simulink model "MVB"  (R2013b)
settings: Solver=ode45  StartTime=0.0  StopTime=2e-5  RelTol=1e-3
libraries: simulink x2
settings Model: Creator=qiji  LastModifiedBy=qiji

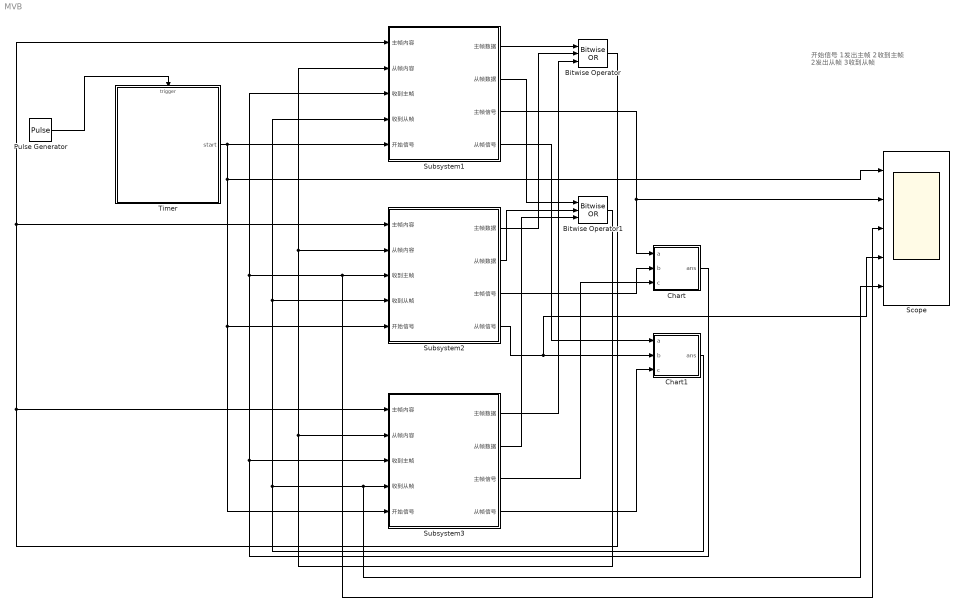
== system MVB ==
  note: 开始信号
      | 1发出主帧
      | 2收到主帧
      | 2发出从帧
      | 3收到从帧
  Bitwise Operator : simulink/Logic and Bit Operations/Bitwise Operator  logicop=OR  UseBitMask=off  NumInputPorts=3  BitMask=bin2dec('11011001')  BitMaskRealWorld=Stored Integer
  Bitwise Operator1 : simulink/Logic and Bit Operations/Bitwise Operator  logicop=OR  UseBitMask=off  NumInputPorts=3  BitMask=bin2dec('11011001')  BitMaskRealWorld=Stored Integer
  Chart : Stateflow chart  TreatAsAtomicUnit=on
  Chart1 : Stateflow chart  TreatAsAtomicUnit=on
  Pulse Generator : DiscretePulseGenerator  PulseType=Time based  Period=1e-7  PulseWidth=50
  Scope : Scope  NumInputPorts=5
      settings: YMin=-5~-5~-5~-5~-5  YMax=5~5~5~5~5
  Subsystem1 : Subsystem
  Subsystem2 : Subsystem
  Subsystem3 : Subsystem
  Timer : Stateflow chart  TreatAsAtomicUnit=on
  wires:
  Pulse Generator/1 -> Timer/Trigger
  Timer/1(start) -> Scope/1, Subsystem3/5(开始信号), Subsystem2/5(开始信号), Subsystem1/5(开始信号)
  Subsystem1/1(主帧数据) -> Bitwise Operator/1
  Subsystem2/1(主帧数据) -> Bitwise Operator/2
  Subsystem3/1(主帧数据) -> Bitwise Operator/3
  Bitwise Operator/1 -> Subsystem1/1(主帧内容), Subsystem2/1(主帧内容), Subsystem3/1(主帧内容)
  Chart/1(ans) -> Subsystem3/3(收到主帧), Subsystem1/3(收到主帧), Scope/3, Subsystem2/3(收到主帧)
  Chart1/1(ans) -> Subsystem2/4(收到从帧), Subsystem1/4(收到从帧), Scope/5, Subsystem3/4(收到从帧)
  Subsystem1/2(从帧数据) -> Bitwise Operator1/1
  Subsystem2/2(从帧数据) -> Bitwise Operator1/2
  Subsystem3/2(从帧数据) -> Bitwise Operator1/3
  Bitwise Operator1/1 -> Subsystem3/2(从帧内容), Subsystem1/2(从帧内容), Subsystem2/2(从帧内容)
  Subsystem1/3(主帧信号) -> Scope/2, Chart/1(a)
  Subsystem2/3(主帧信号) -> Chart/2(b)
  Subsystem3/3(主帧信号) -> Chart/3(c)
  Subsystem1/4(从帧信号) -> Chart1/1(a)
  Subsystem2/4(从帧信号) -> Scope/4, Chart1/2(b)
  Subsystem3/4(从帧信号) -> Chart1/3(c)

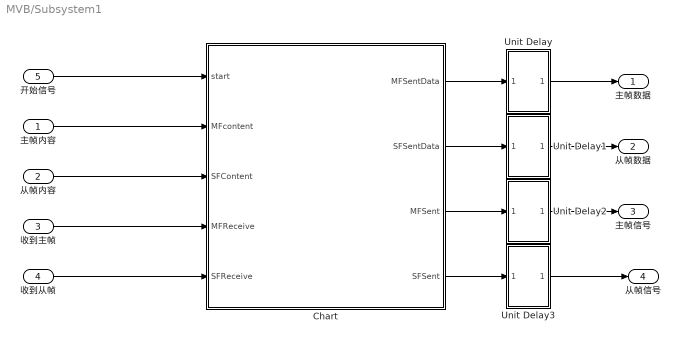
== system MVB/Subsystem1 ==
  主帧内容 : Inport
  从帧内容 : Inport  Port=2
  收到主帧 : Inport  Port=3
  收到从帧 : Inport  Port=4
  开始信号 : Inport  Port=5
  Chart : Stateflow chart  TreatAsAtomicUnit=on
  Unit Delay : Subsystem
  Unit Delay1 : Subsystem
  Unit Delay2 : Subsystem
  Unit Delay3 : Subsystem
  主帧数据 : Outport
  从帧数据 : Outport  Port=2
  主帧信号 : Outport  Port=3
  从帧信号 : Outport  Port=4
  wires:
  从帧内容/1 -> Chart/3(SFContent)
  收到主帧/1 -> Chart/4(MFReceive)
  收到从帧/1 -> Chart/5(SFReceive)
  Chart/2(SFSentData) -> Unit Delay1/1(In1)
  主帧内容/1 -> Chart/2(MFcontent)
  Chart/1(MFSentData) -> Unit Delay/1(In1)
  Chart/4(SFSent) -> Unit Delay3/1(In1)
  Chart/3(MFSent) -> Unit Delay2/1(In1)
  开始信号/1 -> Chart/1(start)
  Unit Delay/1(Out1) -> 主帧数据/1
  Unit Delay1/1(Out1) -> 从帧数据/1
  Unit Delay2/1(Out1) -> 主帧信号/1
  Unit Delay3/1(Out1) -> 从帧信号/1

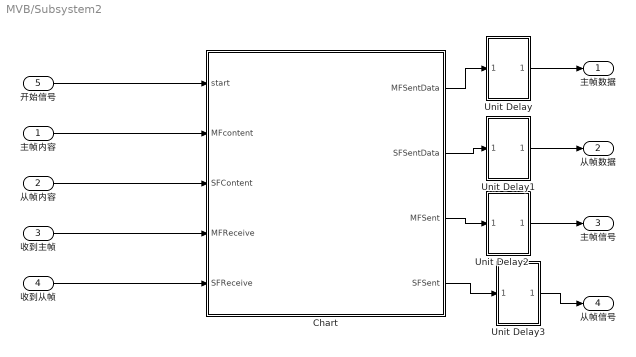
== system MVB/Subsystem2 ==
  主帧内容 : Inport
  从帧内容 : Inport  Port=2
  收到主帧 : Inport  Port=3
  收到从帧 : Inport  Port=4
  开始信号 : Inport  Port=5
  Chart : Stateflow chart  TreatAsAtomicUnit=on
  Unit Delay : Subsystem
  Unit Delay1 : Subsystem
  Unit Delay2 : Subsystem
  Unit Delay3 : Subsystem
  主帧数据 : Outport
  从帧数据 : Outport  Port=2
  主帧信号 : Outport  Port=3
  从帧信号 : Outport  Port=4
  wires:
  从帧内容/1 -> Chart/3(SFContent)
  收到主帧/1 -> Chart/4(MFReceive)
  收到从帧/1 -> Chart/5(SFReceive)
  Chart/2(SFSentData) -> Unit Delay1/1(In1)
  主帧内容/1 -> Chart/2(MFcontent)
  Chart/1(MFSentData) -> Unit Delay/1(In1)
  Chart/4(SFSent) -> Unit Delay3/1(In1)
  Chart/3(MFSent) -> Unit Delay2/1(In1)
  开始信号/1 -> Chart/1(start)
  Unit Delay/1(Out1) -> 主帧数据/1
  Unit Delay1/1(Out1) -> 从帧数据/1
  Unit Delay2/1(Out1) -> 主帧信号/1
  Unit Delay3/1(Out1) -> 从帧信号/1

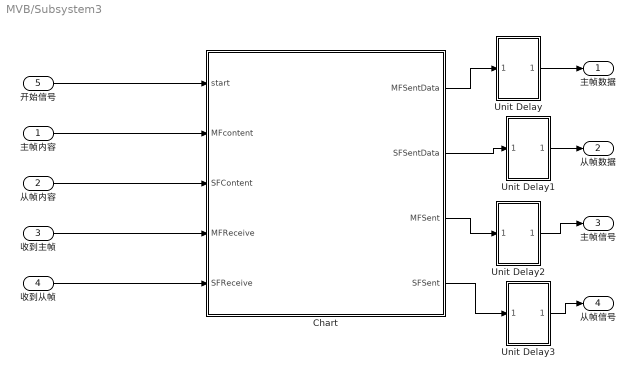
== system MVB/Subsystem3 ==
  主帧内容 : Inport
  从帧内容 : Inport  Port=2
  收到主帧 : Inport  Port=3
  收到从帧 : Inport  Port=4
  开始信号 : Inport  Port=5
  Chart : Stateflow chart  TreatAsAtomicUnit=on
  Unit Delay : Subsystem
  Unit Delay1 : Subsystem
  Unit Delay2 : Subsystem
  Unit Delay3 : Subsystem
  主帧数据 : Outport
  从帧数据 : Outport  Port=2
  主帧信号 : Outport  Port=3
  从帧信号 : Outport  Port=4
  wires:
  从帧内容/1 -> Chart/3(SFContent)
  收到主帧/1 -> Chart/4(MFReceive)
  收到从帧/1 -> Chart/5(SFReceive)
  Chart/2(SFSentData) -> Unit Delay1/1(In1)
  主帧内容/1 -> Chart/2(MFcontent)
  Chart/1(MFSentData) -> Unit Delay/1(In1)
  Chart/4(SFSent) -> Unit Delay3/1(In1)
  Chart/3(MFSent) -> Unit Delay2/1(In1)
  开始信号/1 -> Chart/1(start)
  Unit Delay/1(Out1) -> 主帧数据/1
  Unit Delay1/1(Out1) -> 从帧数据/1
  Unit Delay2/1(Out1) -> 主帧信号/1
  Unit Delay3/1(Out1) -> 从帧信号/1

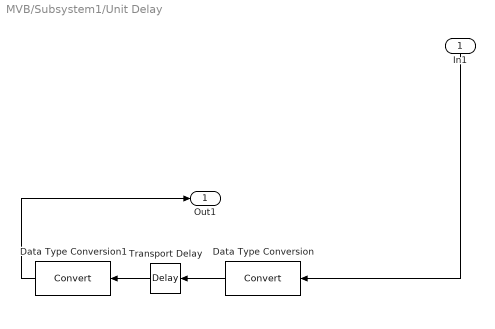
== system MVB/Subsystem1/Unit Delay ==
  In1 : Inport
  Data Type Conversion : DataTypeConversion
  Data Type Conversion1 : DataTypeConversion
  Transport Delay : TransportDelay  DelayTime=1e-7
  Out1 : Outport
  wires:
  In1/1 -> Data Type Conversion/1
  Data Type Conversion/1 -> Transport Delay/1
  Transport Delay/1 -> Data Type Conversion1/1
  Data Type Conversion1/1 -> Out1/1

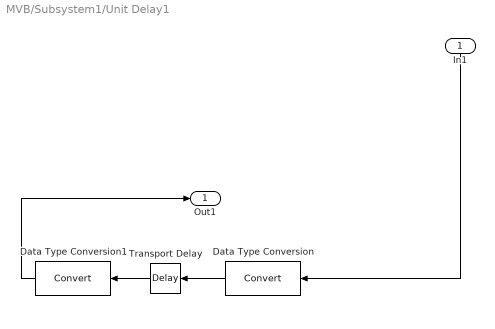
== system MVB/Subsystem1/Unit Delay1 ==
  In1 : Inport
  Data Type Conversion : DataTypeConversion
  Data Type Conversion1 : DataTypeConversion
  Transport Delay : TransportDelay  DelayTime=1e-7
  Out1 : Outport
  wires:
  In1/1 -> Data Type Conversion/1
  Data Type Conversion/1 -> Transport Delay/1
  Transport Delay/1 -> Data Type Conversion1/1
  Data Type Conversion1/1 -> Out1/1

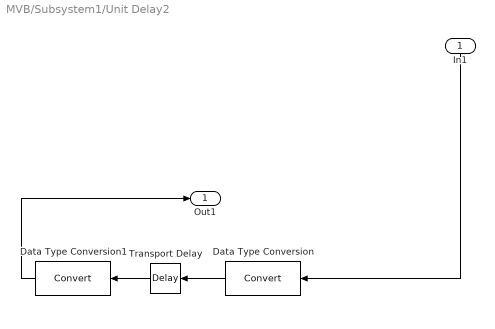
== system MVB/Subsystem1/Unit Delay2 ==
  In1 : Inport
  Data Type Conversion : DataTypeConversion
  Data Type Conversion1 : DataTypeConversion
  Transport Delay : TransportDelay  DelayTime=1e-7
  Out1 : Outport
  wires:
  In1/1 -> Data Type Conversion/1
  Data Type Conversion/1 -> Transport Delay/1
  Transport Delay/1 -> Data Type Conversion1/1
  Data Type Conversion1/1 -> Out1/1

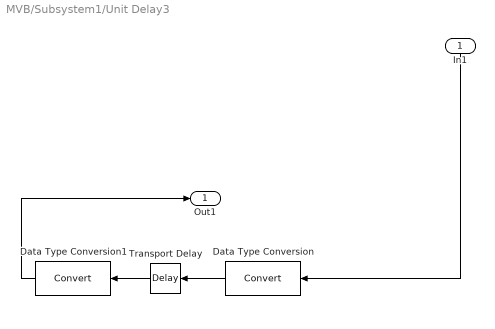
== system MVB/Subsystem1/Unit Delay3 ==
  In1 : Inport
  Data Type Conversion : DataTypeConversion
  Data Type Conversion1 : DataTypeConversion
  Transport Delay : TransportDelay  DelayTime=1e-7
  Out1 : Outport
  wires:
  In1/1 -> Data Type Conversion/1
  Data Type Conversion/1 -> Transport Delay/1
  Transport Delay/1 -> Data Type Conversion1/1
  Data Type Conversion1/1 -> Out1/1

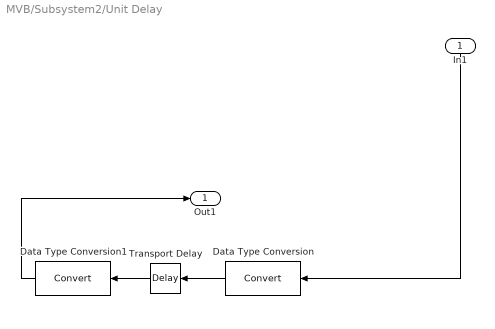
== system MVB/Subsystem2/Unit Delay ==
  In1 : Inport
  Data Type Conversion : DataTypeConversion
  Data Type Conversion1 : DataTypeConversion
  Transport Delay : TransportDelay  DelayTime=1e-7
  Out1 : Outport
  wires:
  In1/1 -> Data Type Conversion/1
  Data Type Conversion/1 -> Transport Delay/1
  Transport Delay/1 -> Data Type Conversion1/1
  Data Type Conversion1/1 -> Out1/1

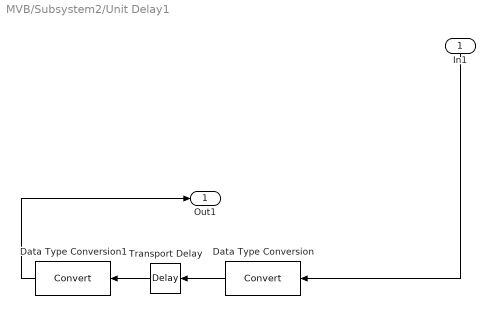
== system MVB/Subsystem2/Unit Delay1 ==
  In1 : Inport
  Data Type Conversion : DataTypeConversion
  Data Type Conversion1 : DataTypeConversion
  Transport Delay : TransportDelay  DelayTime=1e-7
  Out1 : Outport
  wires:
  In1/1 -> Data Type Conversion/1
  Data Type Conversion/1 -> Transport Delay/1
  Transport Delay/1 -> Data Type Conversion1/1
  Data Type Conversion1/1 -> Out1/1

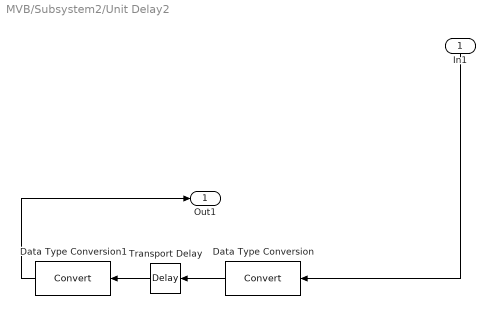
== system MVB/Subsystem2/Unit Delay2 ==
  In1 : Inport
  Data Type Conversion : DataTypeConversion
  Data Type Conversion1 : DataTypeConversion
  Transport Delay : TransportDelay  DelayTime=1e-7
  Out1 : Outport
  wires:
  In1/1 -> Data Type Conversion/1
  Data Type Conversion/1 -> Transport Delay/1
  Transport Delay/1 -> Data Type Conversion1/1
  Data Type Conversion1/1 -> Out1/1

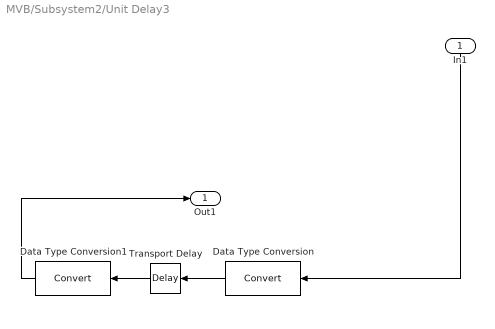
== system MVB/Subsystem2/Unit Delay3 ==
  In1 : Inport
  Data Type Conversion : DataTypeConversion
  Data Type Conversion1 : DataTypeConversion
  Transport Delay : TransportDelay  DelayTime=1e-7
  Out1 : Outport
  wires:
  In1/1 -> Data Type Conversion/1
  Data Type Conversion/1 -> Transport Delay/1
  Transport Delay/1 -> Data Type Conversion1/1
  Data Type Conversion1/1 -> Out1/1

== system MVB/Subsystem3/Unit Delay ==
  In1 : Inport
  Data Type Conversion : DataTypeConversion
  Data Type Conversion1 : DataTypeConversion
  Transport Delay : TransportDelay  DelayTime=1e-7
  Out1 : Outport
  wires:
  In1/1 -> Data Type Conversion/1
  Data Type Conversion/1 -> Transport Delay/1
  Transport Delay/1 -> Data Type Conversion1/1
  Data Type Conversion1/1 -> Out1/1

== system MVB/Subsystem3/Unit Delay1 ==
  In1 : Inport
  Data Type Conversion : DataTypeConversion
  Data Type Conversion1 : DataTypeConversion
  Transport Delay : TransportDelay  DelayTime=1e-7
  Out1 : Outport
  wires:
  In1/1 -> Data Type Conversion/1
  Data Type Conversion/1 -> Transport Delay/1
  Transport Delay/1 -> Data Type Conversion1/1
  Data Type Conversion1/1 -> Out1/1

== system MVB/Subsystem3/Unit Delay2 ==
  In1 : Inport
  Data Type Conversion : DataTypeConversion
  Data Type Conversion1 : DataTypeConversion
  Transport Delay : TransportDelay  DelayTime=1e-7
  Out1 : Outport
  wires:
  In1/1 -> Data Type Conversion/1
  Data Type Conversion/1 -> Transport Delay/1
  Transport Delay/1 -> Data Type Conversion1/1
  Data Type Conversion1/1 -> Out1/1

== system MVB/Subsystem3/Unit Delay3 ==
  In1 : Inport
  Data Type Conversion : DataTypeConversion
  Data Type Conversion1 : DataTypeConversion
  Transport Delay : TransportDelay  DelayTime=1e-7
  Out1 : Outport
  wires:
  In1/1 -> Data Type Conversion/1
  Data Type Conversion/1 -> Transport Delay/1
  Transport Delay/1 -> Data Type Conversion1/1
  Data Type Conversion1/1 -> Out1/1

== stateflow chart MVB/Timer ==
  state startTimer
  state cycle
  (default) -> startTimer
  startTimer -> cycle : {
      | cycleCount = 1000;
      | }
  (junction 5) -> cycle [order 2]
  (junction 5) -> cycle [order 1] : [cycleCount>=1000]{cycleCount=0;start = 1;}
  cycle -> (junction 5) : pulse
      | {
      | cycleCount++;
      | start = 0;
      |  }
  data: cycleCount local uint32; start output uint8
  events: pulse input RISING_EDGE_EVENT

== stateflow chart MVB/Subsystem1/Chart ==
  state startState
  state SEquipment
    state waitMF
    state judge
    state destin
    state source
    state waitSF
    state sendSF
    state checkSF
    state judgeSF
    state storeSF
    (default) -> waitMF
    waitMF -> judge : [MFReceive == 1]
        | {
        | MFaddr = MFcontent;
        | }
    judge -> destin [order 3]
    judge -> source [order 1] : [MFaddr == (logicAddr >> 12 )]
    destin -> waitSF : {
        | SFCount = 0;
        | }
    source -> sendSF : {
        | SFSent = 1;
        | SFSentData = getCongData();
        | Wait4us = 0;
        | }
    waitSF -> judgeSF [order 1] : [SFCount <= 42]
        | {
        | SFCount++;
        | }
    waitSF -> checkSF [order 2]
    judgeSF -> waitSF [order 2]
    (junction 178) -> sendSF
    sendSF -> (junction 178) [order 1] : [Wait4us <= 4]
        | {
        | Wait4us++;
        | }
    checkSF -> storeSF [order 1] : [SFReceive == 1]
        | {
        | SFCount = 0;
        | store[storeIndex] = SFContent;
        | storeIndex++;
        | }
    judgeSF -> checkSF [order 1] : [SFReceive==1]
  state MEquipment
    state waitStart
    state beforeSend
    state sendMF
    (default) -> waitStart
    waitStart -> beforeSend : [start==1]
        | {
        | MFSent = 0;
        | SFSent = 0;
        | }
    beforeSend -> MEquipment [order 2]
    beforeSend -> sendMF [order 1] : [MFNum>0]
        | {
        | MFSent = 1;
        | MFNum--;
        | MFSentData = MFT[i];
        | }
  note: 从帧和主帧已经发出，
      | 等待下一轮周期
  state r = getAddr(f_code, addr, addrReal) [function]
    (default) -> (junction 59) : {
        | r = addrReal;
        | r += (addr << 12);
        | r += (f_code << 24);
        | }
  state init [function]
    (default) -> (junction 4) : {
        | isMaster[1] = true;
        | isMaster[2] = true;
        | isMaster[3] = false;
        | isMaster[4] = false;
        | MFNum = 2;
        | i=1;
        | MFT[1] = getMF(0, 2);
        | MFT[2] = getMF(0, 3);
        | logicAddr = getAddr(0, 1, 5);
        | store[1] = 11;
        | store[2] = 22;
        | store[3] = 33;
        | store[4] = 44;
        | store[5] = 55;
        | store[6] = 66;
        | storeIndex = 7;
        | MFSent = 0;
        | SFSent = 0;
        | }
  state r = getMF(f_code, addr) [function]
    (default) -> (junction 18) : {
        | r = f_code<<12;
        | r += addr;
        | }
  state r = getCongData [function]
    (default) -> (junction 80) : {
        | r = store[logicAddr & 4095]
        | }
  (default) -> startState : {init();}
  startState -> SEquipment [order 2] : {
      | MFSent = 0;
      | SFSent = 0;
      | }
  startState -> MEquipment [order 1] : [isMaster[i]==true]
  (junction 139) -> startState : {
      | i++;
      | }
  sendMF -> (junction 139) : {
      | MFSent = 0;
      | MFSentData = 0;
      | }
  storeSF -> (junction 139)
  sendSF -> (junction 139) [order 2] : {
      | SFSent = 0;
      | }
  checkSF -> (junction 139) [order 2]
  judge -> MEquipment [order 2] : [isMaster[i]==true]
  data: r function_output double; f_code function_input double; addr function_input double; addrReal function_input double; f_code function_input double; addr function_input double; r function_output double; r function_output double; isMaster local boolean size=100; start input uint8; MFT local uint32 size=10; MFNum local uint8; i local uint8; MFSentData output uint32; MFcontent input uint32; logicAddr local uint32; store local uint32 size=100; SFSentData output uint32; storeIndex local uint32; SFContent input uint32; MFaddr local uint32; MFSent output uint8; SFSent output uint8; MFReceive input uint8; SFReceive input uint8; Wait4us local uint32; SFCount local uint32

== stateflow chart MVB/Subsystem2/Chart ==
  state startState
  state SEquipment
    state waitMF
    state judge
    state destin
    state source
    state waitSF
    state sendSF
    state checkSF
    state storeSF
    (default) -> waitMF
    waitMF -> judge : [MFReceive == 1]
        | {
        | MFaddr = MFcontent;
        | }
    judge -> destin [order 3]
    judge -> source [order 1] : [MFaddr == (logicAddr >> 12 )]
    source -> sendSF : {
        | SFSent = 1;
        | SFSentData = getCongData();
        | Wait4us=0;
        | }
    destin -> waitSF : {
        | SFCount = 0;
        | }
    waitSF -> checkSF [order 2]
    (junction 174) -> sendSF
    sendSF -> (junction 174) [order 1] : [Wait4us<=4]
        | {
        | Wait4us++;
        | }
    checkSF -> storeSF [order 1] : [SFReceive == 1]
        | {
        | SFCount = 0;
        | store[storeIndex] = SFContent;
        | storeIndex++;
        | }
  state MEquipment
    state waitStart
    state beforeSend
    state sendMF
    (default) -> waitStart
    waitStart -> beforeSend : [start==1]
        | {
        | MFSent = 0;
        | SFSent = 0;
        | }
    beforeSend -> MEquipment [order 2]
    beforeSend -> sendMF [order 1] : [MFNum>0]
        | {
        | MFSent = 1;
        | MFNum--;
        | MFSentData = MFT[i];
        | }
  note: 从帧和主帧已经发出，
      | 等待下一轮周期
  state judgeSF
  state r = getAddr(f_code, addr, addrReal) [function]
    (default) -> (junction 59) : {
        | r = addrReal;
        | r += (addr << 12);
        | r += (f_code << 24);
        | }
  state init [function]
    (default) -> (junction 4) : {
        | isMaster[1] = false;
        | isMaster[2] = false;
        | isMaster[3] = true;
        | isMaster[4] = false;
        | MFNum = 2;
        | i=1;
        | MFT[3] = getMF(0, 1);
        | logicAddr = getAddr(0, 2, 3);
        | store[1] = 11;
        | store[2] = 22;
        | store[3] = 33;
        | store[4] = 44;
        | store[5] = 55;
        | store[6] = 66;
        | storeIndex = 7;
        | MFSent = 0;
        | SFSent = 0;
        | }
  state r = getMF(f_code, addr) [function]
    (default) -> (junction 18) : {
        | r = f_code<<12;
        | r += addr;
        | }
  state r = getCongData [function]
    (default) -> (junction 80) : {
        | r = store[logicAddr & 4095]
        | }
  (default) -> startState : {init();}
  startState -> SEquipment [order 2] : {
      | MFSent = 0;
      | SFSent  =0;
      | }
  startState -> MEquipment [order 1] : [isMaster[i]==true]
  (junction 139) -> startState : {
      | i++;
      | }
  sendMF -> (junction 139) : {
      | MFSent = 0;
      | MFSentData = 0;
      | }
  storeSF -> (junction 139)
  sendSF -> (junction 139) [order 2] : {
      | SFSent = 0;
      | }
  checkSF -> (junction 139) [order 2]
  judge -> MEquipment [order 2] : [isMaster[i]==true]
  waitSF -> judgeSF [order 1] : [SFCount <= 42]
      | {
      | SFCount++;
      | }
  judgeSF -> waitSF [order 2]
  judgeSF -> checkSF [order 1] : [SFReceive == 1]
  data: r function_output double; f_code function_input double; addr function_input double; addrReal function_input double; f_code function_input double; addr function_input double; r function_output double; r function_output double; isMaster local boolean size=100; start input uint8; MFT local uint32 size=10; MFNum local uint8; i local uint8; MFSentData output uint32; MFcontent input uint32; logicAddr local uint32; store local uint32 size=100; SFSentData output uint32; storeIndex local uint32; SFContent input uint32; MFaddr local uint32; SFCount local uint32; MFSent output uint8; SFSent output uint8; MFReceive input uint8; SFReceive input uint8; Wait4us local uint32

== stateflow chart MVB/Subsystem3/Chart ==
  state startState
  state SEquipment
    state waitMF
    state judge
    state destin
    state source
    state waitSF
    state sendSF
    state checkSF
    state storeSF
    (default) -> waitMF
    waitMF -> judge : [MFReceive == 1]
        | {
        | MFaddr = MFcontent;
        | }
    judge -> destin [order 3]
    judge -> source [order 1] : [MFaddr == (logicAddr >> 12 )]
    source -> sendSF : {
        | SFSent = 1;
        | SFSentData = getCongData();
        | Wait4us = 0;
        | }
    destin -> waitSF : {
        | SFCount = 0;
        | }
    waitSF -> checkSF [order 2]
    (junction 149) -> sendSF
    sendSF -> (junction 149) [order 1] : [Wait4us<=4]
        | {
        | Wait4us++;
        | }
    checkSF -> storeSF [order 1] : [SFReceive == 1]
        | {
        | SFCount = 0;
        | store[storeIndex] = SFContent;
        | storeIndex++;
        | }
  state MEquipment
    state waitStart
    state beforeSend
    state sendMF
    (default) -> waitStart
    waitStart -> beforeSend : [start==1]
        | {
        | MFSent = 0;
        | SFSent = 0;
        | }
    beforeSend -> MEquipment [order 2]
    beforeSend -> sendMF [order 1] : [MFNum>0]
        | {
        | MFSent = 1;
        | MFNum--;
        | MFSentData = MFT[i];
        | }
  note: 从帧和主帧已经发出，
      | 等待下一轮周期
  state judgeSF
  state r = getAddr(f_code, addr, addrReal) [function]
    (default) -> (junction 59) : {
        | r = addrReal;
        | r += (addr << 12);
        | r += (f_code << 24);
        | }
  state init [function]
    (default) -> (junction 4) : {
        | isMaster[1] = false;
        | isMaster[2] = false;
        | isMaster[3] = false;
        | isMaster[4] = false;
        | MFNum = 2;
        | i=1;
        | MFT[1] = getMF(0, 1);
        | MFT[2] = getMF(0, 1);
        | logicAddr = getAddr(0, 3, 5);
        | store[1] = 11;
        | store[2] = 22;
        | store[3] = 33;
        | store[4] = 44;
        | store[5] = 55;
        | store[6] = 66;
        | storeIndex = 7;
        | MFSent = 0;
        | SFSent = 0;
        | }
  state r = getMF(f_code, addr) [function]
    (default) -> (junction 18) : {
        | r = f_code<<12;
        | r += addr;
        | }
  state r = getCongData [function]
    (default) -> (junction 80) : {
        | r = store[logicAddr & 4095]
        | }
  (default) -> startState : {init();}
  startState -> SEquipment [order 2] : {
      | SFSent = 0;
      | MFSent = 0;
      | }
  startState -> MEquipment [order 1] : [isMaster[i]==true]
  (junction 130) -> startState : {
      | i++;
      | }
  sendMF -> (junction 130) : {
      | MFSent = 0;
      | MFSentData = 0;
      | }
  storeSF -> (junction 130)
  checkSF -> (junction 130) [order 2]
  sendSF -> (junction 130) [order 2] : {
      | SFSent = 0;
      | }
  judge -> MEquipment [order 2] : [isMaster[i]==true]
  waitSF -> judgeSF [order 1] : [SFCount <= 42]
      | {
      | SFCount++;
      | }
  judgeSF -> waitSF [order 2]
  judgeSF -> checkSF [order 1] : [SFReceive == 1]
  data: r function_output double; f_code function_input double; addr function_input double; addrReal function_input double; f_code function_input double; addr function_input double; r function_output double; r function_output double; isMaster local boolean size=100; start input uint8; MFT local uint32 size=10; MFNum local uint8; i local uint8; MFSentData output uint32; MFcontent input uint32; logicAddr local uint32; store local uint32 size=100; SFSentData output uint32; storeIndex local uint32; SFContent input uint32; MFaddr local uint32; MFSent output uint8; SFSent output uint8; MFReceive input uint8; SFReceive input uint8; Wait4us local uint32; SFCount local uint32

== stateflow chart MVB/Chart ==
  state judge
  state NULL
  state OK
  note: ?
  note: ?
  note: ?
  note: ?
  (default) -> judge
  judge -> NULL [order 2] : [(a+b+c)==0]
      | {
      | ans = 0;
      | }
  judge -> OK [order 1] : [(a+b+c)==1]
      | {
      | ans = 1;
      | }
  OK -> NULL : [a+b+c==0]
      | {
      | ans=0;
      | }
  NULL -> OK : [a+b+c==1]
      | {
      | ans=1;
      | }
  data: ans output uint8; a input uint8; b input uint8; c input uint8

== stateflow chart MVB/Chart1 ==
  state judge
  state NULL
  state OK
  note: ?
  note: ?
  note: ?
  note: ?
  (default) -> judge
  judge -> NULL [order 2] : [(a+b+c)==0]
      | {
      | ans = 0;
      | }
  judge -> OK [order 1] : [(a+b+c)==1]
      | {
      | ans = 1;
      | }
  OK -> NULL : [(a+b+c)==0]
      | {
      | ans=0;
      | }
  NULL -> OK : [(a+b+c)==1]
      | {
      | ans=1;
      | }
  data: ans output uint8; a input uint8; b input uint8; c input uint8
